simulink model "PassengerCar"  (R2019b)
settings: Solver=ode1  StartTime=0  StopTime=25  FixedStep=1.0000000000000000e-003  RelTol=1e-3
InitFcn:
  | sampleTime = str2double(get_param(bdroot, 'FixedStep'));
undefined symbols (not defined in the file or in its folder): AccPedalPos, BrakePedalPos, BrakeSwitch, DiscIntNeverNeededParam, DYNA4, EngSpd, IgnitionSwitch, InitialGear, InitialSpeed, IntendedEngTrq, LeftIndicator, MainBrakePress, MaxGear, MDL, MinGear, RefAcc, RefLane, RefLatPos, RefPath, RefPathCurv, RefSpd, RefSpdPreview, RefSpdRetrospect, RightIndicator, SteeringWheelAng, SteeringWheelTrq, UserDefinedRefValue, vm_const
libraries: UtilitiesLibrary x31, simulink x18, WheelSystemModules x13, LongitudinalControllerModules x13, LateralControllerModules x7, AnimationBusselectorModules x5, EnvironmentModules x5, BasicEngineControlModules x5, MiscellaneousControlModules x5, Animation3Modules x4, AuxiliariesModules x4, TireModules x4
(part 4 of 39)

== system PassengerCar/Traffic ==
  fromCTRL : Inport
  fromVehicle : Inport  Port=2
  DynaComponentInfo : Subsystem  Tag=DynaComponentInfo
      mask init:
      | data= get_param(gcb, 'UserData');
      settings: OpenFcn=DYNA4.ModelHandling.Component.ShowEditComponentInformationDialog(gcb);
      mask Display: disp(['Type = ', data.type, '\nGroup = ', data.group, '\nName = ', data.name ])
  Terminator : Terminator
  Terminator1 : Terminator
  TrafficOutputs : Subsystem
  Traffic : Outport  VectorParamsAs1DForOutWhenUnconnected=off
  wires:
  TrafficOutputs/1(Traffic) -> Traffic/1
  fromCTRL/1 -> Terminator/1
  fromVehicle/1 -> Terminator1/1

== system PassengerCar/Trailer ==
  fromCTRL : Inport
  fromVehicle : Inport  Port=2
  DynaComponentInfo : Subsystem  Tag=DynaComponentInfo
      mask init:
      | data= get_param(gcb, 'UserData');
      settings: OpenFcn=DYNA4.ModelHandling.Component.ShowEditComponentInformationDialog(gcb);
      mask Display: disp(['Type = ', data.type, '\nGroup = ', data.group, '\nName = ', data.name ])
  Terminator1 : Terminator
  Terminator4 : Terminator
  TrailerOutput : ReducedChassisModules/TrailerOutput  SystemSampleTime=-1  Latency=0  AutoFrameSizeCalculation=off
  Trailer : Outport  VectorParamsAs1DForOutWhenUnconnected=off
  wires:
  fromCTRL/1 -> Terminator4/1
  fromVehicle/1 -> Terminator1/1
  TrailerOutput/1 -> Trailer/1

== system PassengerCar/Vehicle ==
  fromCTRL : Inport
  fromTrailer : Inport  Port=2
  fromEnvironment : Inport  Port=3
  AnimationContentVehicle : Animation3Modules/AnimationContentVehicle  SystemSampleTime=-1  Latency=0  AutoFrameSizeCalculation=off
  Auxiliaries : Subsystem  Tag=vedynaEngineMask
  BrakeSystem : Subsystem  Tag=vedynaEngineMask
  Chassis : Subsystem  Tag=COMPONENT_CHASSIS
  CoolingSystem : Subsystem
  DriverInformationVehicle : DriverInformationModules/DriverInformationVehicle  DATA_NODE=MDL.Vehicle.DriverInformationVehicle  EngInrt=MDL.Vehicle.DriverInformationVehicle.EngInrt  OverallMass=MDL.Vehicle.DriverInformationVehicle.OverallMass  CoGPos=MDL.Vehicle.DriverInformationVehicle.CoGPos  FrontRearWheelBase=MDL.Vehicle.DriverInformationVehicle.FrontRearWheelBase  YawInrt=MDL.Vehicle.DriverInformationVehicle.YawInrt  FrontSteeringRatio=MDL.Vehicle.DriverInformationVehicle.FrontSteeringRatio  MaxLeftSteeringWheelAng=MDL.Vehicle.DriverInformationVehicle.MaxLeftSteeringWheelAng  MaxRightSteeringWheelAng=MDL.Vehicle.DriverInformationVehicle.MaxRightSteeringWheelAng  TransmissionType=MDL.Vehicle.DriverInformationVehicle.TransmissionType  NumFwdGears=MDL.Vehicle.DriverInformationVehicle.NumFwdGears  FrontTireUnloadedRadius=MDL.Vehicle.DriverInformationVehicle.FrontTireUnloadedRadius  RearTireUnloadedRadius=MDL.Vehicle.DriverInformationVehicle.RearTireUnloadedRadius  WheelRotAxisInrt=MDL.Vehicle.DriverInformationVehicle.WheelRotAxisInrt  MaxMainBrakePress=MDL.Vehicle.DriverInformationVehicle.MaxMainBrakePress  MaxDec=MDL.Vehicle.DriverInformationVehicle.MaxDec  LongAeroDragCoeff=MDL.Vehicle.DriverInformationVehicle.LongAeroDragCoeff  nShiftECU=MDL.Vehicle.DriverInformationVehicle.nShiftECU  FrontAxleLatStiff=MDL.Vehicle.DriverInformationVehicle.FrontAxleLatStiff  RearAxleLatStiff=MDL.Vehicle.DriverInformationVehicle.RearAxleLatStiff  EngTrqController=MDL.Vehicle.DriverInformationVehicle.EngTrqController
  Drivetrain : Subsystem  Tag=COMPONENT_DRIVETRAIN
  DynaComponentInfo : Subsystem  Tag=DynaComponentInfo
      mask init:
      | data= get_param(gcb, 'UserData');
      settings: OpenFcn=DYNA4.ModelHandling.Component.ShowEditComponentInformationDialog(gcb);
      mask Display: disp(['Type = ', data.type, '\nGroup = ', data.group, '\nName = ', data.name ])
  ElectricalSystem : Subsystem
  Engine : Subsystem  Tag=COMPONENT_ENGINE
  VehicleOutput : Subsystem  Tag=TESIS DYNAware Interface Block  mask{NeedsUpdate=off, SignalInfo=|}
      mask SignalInfo=|
      | {
      |   "Version": "4.6",
      |   "MuxedOutputBusName": "Vehicle",
      |   "MuxedInputBusName": "input",
      |   "MuxedInputSelected": false,
      |   "MuxedOutputSelected": true,
      |   "SignalData": [
      |     {
      |       "initialValue": "0.0",
      |       "name": "Auxiliaries",
      |       "comment": "",
      |       "minString": "",
      |       "maxString": "",
      |       "width": -1,
      |       "dataType": 0,
      |       "signalType": 1,
      |       "createSignal": false,
      |       "outputName": "Auxiliaries",
      |       "generateSignalAccessBlock": false,
      |       "accessId": "$(parentId).$(blockName).$(outputName)"
      |     },
      |     {
      |       "initialValue": "0.0",
      |       "name": "BrakeSystem",
      |       "comment": "",
      |       "minString": "",
      |       "maxString": "",
      |       "width": -1,
      |       "dataType": 0,
      |       "signalType": 1,
      |       "createSignal": false,
      |       "outputName": "BrakeSystem",
      |       "generateSignalAccessBlock": false,
      |       "accessId": "$(parentId).$(blockName).$(outputName)"
      |     },
      |     {
      |       "initialValue": "0.0",
      |       "name": "Chassis",
      |       "comment": "",
      |       "minString": "",
      |       "maxString": "",
      |       "width": -1,
      |       "dataType": 0,
      |       "signalType": 1,
      |       "createSignal": false,
      |       "outputName": "Chassis",
      |       "generateSignalAccessBlock": false,
      |       "accessId": "$(parentId).$(blockName).$(outputName)"
      |     },
      |     {
      |       "initialValue": "0.0",
      |       "name": "Drivetrain",
      |       "comment": "",
      |       "minString": "",
      |       "maxString": "",
      |       "width": -1,
      |       "dataType": 0,
      |       "signalType": 1,
      |       "createSignal": false,
      |       "outputName": "Drivetrain",
      |       "generateSignalAccessBlock": false,
      |       "accessId": "$(parentId).$(blockName).$(outputName)"
      |     },
      |     {
      |       "initialValue": "0.0",
      |       "name": "ElectricalSystem",
      |       "comment": "",
      |       "minString": "",
      |       "maxString": "",
      |       "width": -1,
      |       "dataType": 0,
      |       "signalType": 1,
      |       "createSignal": false,
      |       "outputName": "ElectricalSystem",
      |       "generateSignalAccessBlock": false,
      |       "accessId": "$(parentId).$(blockName).$(outputName)"
      |     },
      |     {
      |       "initialValue": "0.0",
      |       "name": "Engine",
      |       "comment": "",
      |       "minString": "",
      |       "maxString": "",
      |       "width": -1,
      |       "dataType": 0,
      |       "signalType": 1,
      |       "createSignal": false,
      |       "outputName": "Engine",
      |       "generateSignalAccessBlock": false,
      |       "accessId": "$(parentId).$(blockName).$(outputName)"
      |     },
      |     {
      |       "initialValue": "0.0",
      |       "name": "WheelSystem",
      |       "comment": "",
      |       "minString": "",
      |       "maxString": "",
      |       "width": -1,
      |       "dataType": 0,
      |       "signalType": 1,
      |       "createSignal": false,
      |       "outputName": "WheelSystem",
      |       "generateSignalAccessBlock": false,
      |       "accessId": "$(parentId).$(blockName).$(outputName)"
      |     },
      |     {
      |       "initialValue": "0.0",
      |       "name": "CoolingSystem",
      |       "comment": "",
      |       "minString": "",
      |       "maxString": "",
      |       "width": -1,
      |       "dataType": 0,
      |       "signalType": 1,
      |       "createSignal": false,
      |       "outputName": "CoolingSystem",
      |       "generateSignalAccessBlock": false,
      |       "accessId": "$(parentId).$(blockName).$(outputName)"
      |     },
      |     {
      |       "initialValue": "0.0",
      |       "name": "VehicleRoadInfo",
      |       "comment": "",
      |       "minString": "",
      |       "maxString": "",
      |       "width": -1,
      |       "dataType": 0,
      |       "signalType": 1,
      |       "createSignal": false,
      |       "outputName": "VehicleRoadInfo",
      |       "generateSignalAccessBlock": false,
      |       "accessId": "$(parentId).$(blockName).$(outputName)"
      |     },
      |     {
      |       "initialValue": "0.0",
      |       "name": "VehicleDriverInfo",
      |       "comment": "",
      |       "minString": "",
      |       "maxString": "",
      |       "width": -1,
      |       "dataType": 0,
      |       "signalType": 1,
      |       "createSignal": false,
      |       "outputName": "VehicleDriverInfo",
      |       "generateSignalAccessBlock": false,
      |       "accessId": "$(parentId).$(blockName).$(outputName)"
      |     }
      |   ]
      | }
      mask prompts: NeedsUpdate "Specify, if subsystem content needs to be updated"; SignalInfo "Signal Info (json)"
      mask help: DYNA4 Interface Block Version 4.6
      mask init:
      | blockName = get_param(gcbh, 'Name');
      | parentId = DYNA4.ModelHandling.AccessID.getFromHierarchy(gcbh);
      | TD.InterfaceBlock.ModelCallbacks.GenerateContent(gcb);
      settings: DeleteFcn=TD.InterfaceBlock.ModelCallbacks.CloseGUI( gcbh );  NameChangeFcn=TD.InterfaceBlock.ModelCallbacks.BlockRenamedHandler(gcbh);  OpenFcn=TD.InterfaceBlock.ModelCallbacks.OpenGUI( gcbh );  CloseFcn=TD.InterfaceBlock.ModelCallbacks.CloseGUI( gcbh );
      mask Display:
      | image('InterfaceBlock.png','center');
      | port_label('input',1, 'Auxiliaries');
      | port_label('input',2, 'BrakeSystem');
      | port_label('input',3, 'Chassis');
      | port_label('input',4, 'Drivetrain');
      | port_label('input',5, 'ElectricalSystem');
      | port_label('input',6, 'Engine');
      | port_label('input',7, 'WheelSystem');
      | port_label('input',8, 'CoolingSystem');
      | port_label('input',9, 'VehicleRoadInfo');
      | port_label('input',10, 'VehicleDriverInfo');
      | port_label('output',1, 'Vehicle');
  VehicleRoadInfo : Subsystem
  WheelSystem : Subsystem  Tag=COMPONENT_WHEELSYSTEM
  Vehicle : Outport  VectorParamsAs1DForOutWhenUnconnected=off
  wires:
  DriverInformationVehicle/1 -> VehicleOutput/10(VehicleDriverInfo___UNIQUE_1)
  VehicleRoadInfo/1(VehicleRoadInfo) -> VehicleOutput/9(VehicleRoadInfo___UNIQUE_1)
  CoolingSystem/1(CoolingSystem) -> VehicleOutput/8(CoolingSystem___UNIQUE_1)
  fromTrailer/1 -> Chassis/2(fromTrailer)
  fromEnvironment/1 -> CoolingSystem/6(fromEnvironment), Engine/2(fromEnvironment)
  fromCTRL/1 -> Auxiliaries/1(fromCTRL), Chassis/1(fromCTRL), Drivetrain/1(fromCTRL), ElectricalSystem/1(fromCTRL), DriverInformationVehicle/1, VehicleRoadInfo/1(fromCTRL), CoolingSystem/1(fromCTRL), WheelSystem/1(fromCTRL), Engine/1(fromCTRL), BrakeSystem/1(fromCTRL)
  ElectricalSystem/1(ElectricalSystem) -> CoolingSystem/5(fromElectricalSystem), Engine/5(fromElectricalSystem), Drivetrain/3(fromElectricalSystem), Auxiliaries/3(fromElectricalSystem), VehicleOutput/5(ElectricalSystem___UNIQUE_1)
  VehicleOutput/1(Vehicle___UNIQUE_1) -> Vehicle/1
  BrakeSystem/1(BrakeSystem) -> DriverInformationVehicle/2, WheelSystem/2(fromBrakeSystem), VehicleOutput/2(BrakeSystem___UNIQUE_1)
  Auxiliaries/1(Auxiliaries) -> ElectricalSystem/2(fromAuxiliaries), Drivetrain/2(fromAuxiliaries), VehicleOutput/1(Auxiliaries___UNIQUE_1)
  Chassis/1(Chassis) -> DriverInformationVehicle/3, VehicleRoadInfo/2(fromChassis), CoolingSystem/2(fromChassis), WheelSystem/3(fromChassis), Engine/3(fromChassis), BrakeSystem/2(fromChassis), VehicleOutput/3(Chassis___UNIQUE_1)
  Drivetrain/1(Drivetrain) -> Auxiliaries/2(fromDrivetrain), ElectricalSystem/3(fromDrivetrain), DriverInformationVehicle/4, CoolingSystem/4(fromDrivetrain), WheelSystem/4(fromDrivetrain), Engine/4(fromDrivetrain), VehicleOutput/4(Drivetrain___UNIQUE_1)
  WheelSystem/1(WheelSystem) -> DriverInformationVehicle/6, Drivetrain/5(fromWheelSystem), Chassis/4(fromWheelSystem), BrakeSystem/4(fromWheelSystem), VehicleOutput/7(WheelSystem___UNIQUE_1)
  Engine/1(Engine) -> DriverInformationVehicle/5, CoolingSystem/3(fromEngine), ElectricalSystem/4(fromEngine), Drivetrain/4(fromEngine), Chassis/3(fromEngine), Auxiliaries/4(fromEngine), BrakeSystem/3(fromEngine), VehicleOutput/6(Engine___UNIQUE_1)

== system PassengerCar/VehicleControl ==
  fromCTRL : Inport
  fromTrailer : Inport  Port=2
  fromVehicle : Inport  Port=3
  fromTraffic : Inport  Port=4
  DynaComponentInfo : Subsystem  Tag=DynaComponentInfo
      mask init:
      | data= get_param(gcb, 'UserData');
      settings: OpenFcn=DYNA4.ModelHandling.Component.ShowEditComponentInformationDialog(gcb);
      mask Display: disp(['Type = ', data.type, '\nGroup = ', data.group, '\nName = ', data.name ])
  InitialConditions : Subsystem
  LateralControl : Subsystem  VariantControlMode=Label  Variant=on  LabelModeActiveChoice=EnabledLateralControl
  LongitudinalControl : Subsystem
  Miscellaneous : Subsystem
  TraceMarker : UtilitiesLibrary/DYNA4 Trace Marker  Tag=DYNA4_TRACE_MARKER  SettingType=Standard  PrefixModelBlockID=on  PrefixRootSignalName=off  NamePattern='$(modelBlockID).$(rootSignalName)'
  VehicleControlInputs : Subsystem
  VehicleControlOutput : Subsystem  Tag=TESIS DYNAware Interface Block  mask{NeedsUpdate=off, SignalInfo=|}
      mask SignalInfo=|
      | {
      |   "Version": "4.6",
      |   "MuxedOutputBusName": "VehicleControl",
      |   "MuxedInputBusName": "fromLongitudinalControl",
      |   "MuxedInputSelected": false,
      |   "MuxedOutputSelected": true,
      |   "SignalData": [
      |     {
      |       "initialValue": "0.0",
      |       "name": "InitialConditions",
      |       "comment": "",
      |       "minString": "",
      |       "maxString": "",
      |       "width": -1,
      |       "dataType": 0,
      |       "signalType": 1,
      |       "createSignal": false,
      |       "outputName": "InitialConditions",
      |       "generateSignalAccessBlock": false,
      |       "accessId": "$(parentId).$(blockName).$(outputName)"
      |     },
      |     {
      |       "initialValue": "0.0",
      |       "name": "LongitudinalControl",
      |       "comment": "",
      |       "minString": "",
      |       "maxString": "",
      |       "width": -1,
      |       "dataType": 0,
      |       "signalType": 1,
      |       "createSignal": false,
      |       "outputName": "LongitudinalControl",
      |       "generateSignalAccessBlock": false,
      |       "accessId": "$(parentId).$(blockName).$(outputName)"
      |     },
      |     {
      |       "initialValue": "0.0",
      |       "name": "LateralControl",
      |       "comment": "",
      |       "minString": "",
      |       "maxString": "",
      |       "width": -1,
      |       "dataType": 0,
      |       "signalType": 1,
      |       "createSignal": false,
      |       "outputName": "LateralControl",
      |       "generateSignalAccessBlock": false,
      |       "accessId": "$(parentId).$(blockName).$(outputName)"
      |     },
      |     {
      |       "initialValue": "0.0",
      |       "name": "BrakeHydraulicsControl",
      |       "comment": "",
      |       "minString": "",
      |       "maxString": "",
      |       "width": -1,
      |       "dataType": 0,
      |       "signalType": 1,
      |       "createSignal": false,
      |       "outputName": "BrakeHydraulicsControl",
      |       "generateSignalAccessBlock": false,
      |       "accessId": "$(parentId).$(blockName).$(outputName)"
      |     },
      |     {
      |       "initialValue": "0.0",
      |       "name": "EngineControl",
      |       "comment": "",
      |       "minString": "",
      |       "maxString": "",
      |       "width": -1,
      |       "dataType": 0,
      |       "signalType": 1,
      |       "createSignal": false,
      |       "outputName": "EngineControl",
      |       "generateSignalAccessBlock": false,
      |       "accessId": "$(parentId).$(blockName).$(outputName)"
      |     },
      |     {
      |       "initialValue": "0.0",
      |       "name": "SuspensionTestRigControl",
      |       "comment": "",
      |       "minString": "",
      |       "maxString": "",
      |       "width": -1,
      |       "dataType": 0,
      |       "signalType": 1,
      |       "createSignal": false,
      |       "outputName": "SuspensionTestRigControl",
      |       "generateSignalAccessBlock": false,
      |       "accessId": "$(parentId).$(blockName).$(outputName)"
      |     },
      |     {
      |       "initialValue": "0.0",
      |       "name": "TemperatureControl",
      |       "comment": "",
      |       "minString": "",
      |       "maxString": "",
      |       "width": -1,
      |       "dataType": 0,
      |       "signalType": 1,
      |       "createSignal": false,
      |       "outputName": "TemperatureControl",
      |       "generateSignalAccessBlock": false,
      |       "accessId": "$(parentId).$(blockName).$(outputName)"
      |     },
      |     {
      |       "initialValue": "0.0",
      |       "name": "UserDefinedControl",
      |       "comment": "",
      |       "minString": "",
      |       "maxString": "",
      |       "width": -1,
      |       "dataType": 0,
      |       "signalType": 1,
      |       "createSignal": false,
      |       "outputName": "UserDefinedControl",
      |       "generateSignalAccessBlock": false,
      |       "accessId": "$(parentId).$(blockName).$(outputName)"
      |     }
      |   ]
      | }
      mask prompts: NeedsUpdate "Specify, if subsystem content needs to be updated"; SignalInfo "Signal Info (json)"
      mask help: DYNA4 Interface Block Version 4.6
      mask init:
      | blockName = get_param(gcbh, 'Name');
      | parentId = DYNA4.ModelHandling.AccessID.getFromHierarchy(gcbh);
      | TD.InterfaceBlock.ModelCallbacks.GenerateContent(gcb);
      settings: DeleteFcn=TD.InterfaceBlock.ModelCallbacks.CloseGUI( gcbh );  NameChangeFcn=TD.InterfaceBlock.ModelCallbacks.BlockRenamedHandler(gcbh);  OpenFcn=TD.InterfaceBlock.ModelCallbacks.OpenGUI( gcbh );  CloseFcn=TD.InterfaceBlock.ModelCallbacks.CloseGUI( gcbh );
      mask Display:
      | image('InterfaceBlock.png','center');
      | port_label('input',1, 'InitialConditions');
      | port_label('input',2, 'LongitudinalControl');
      | port_label('input',3, 'LateralControl');
      | port_label('input',4, 'BrakeHydraulicsControl');
      | port_label('input',5, 'EngineControl');
      | port_label('input',6, 'SuspensionTestRigControl');
      | port_label('input',7, 'TemperatureControl');
      | port_label('input',8, 'UserDefinedControl');
      | port_label('output',1, 'VehicleControl');
  VehicleControl : Outport  VectorParamsAs1DForOutWhenUnconnected=off
  wires:
  Miscellaneous/2(EngineControlParams) -> VehicleControlOutput/5(EngineControl___UNIQUE_1)
  Miscellaneous/5(UserDefinedControlParams) -> VehicleControlOutput/8(UserDefinedControl___UNIQUE_1)
  Miscellaneous/4(TemperatureControlParams) -> VehicleControlOutput/7(TemperatureControl___UNIQUE_1)
  Miscellaneous/3(SuspensionTestRigControlParams) -> VehicleControlOutput/6(SuspensionTestRigControl___UNIQUE_1)
  fromTraffic/1 -> VehicleControlInputs/4(fromTraffic)
  fromVehicle/1 -> VehicleControlInputs/2(fromVehicle)
  LongitudinalControl/1(LongitudinalControl) -> VehicleControlOutput/2(LongitudinalControl___UNIQUE_1)
  Miscellaneous/1(BrakeHydraulicsParams) -> VehicleControlOutput/4(BrakeHydraulicsControl___UNIQUE_1)
  LateralControl/1(LateralControl) -> VehicleControlOutput/3(LateralControl___UNIQUE_1)
  VehicleControlOutput/1(VehicleControl___UNIQUE_1) -> VehicleControl/1, TraceMarker/1
  fromCTRL/1 -> InitialConditions/1(fromCTRL), VehicleControlInputs/1(fromCTRL)
  VehicleControlInputs/1(SchedulerAbscissae) -> LateralControl/1(SchedulerAbscissae), LongitudinalControl/1(SchedulerAbscissae)
  VehicleControlInputs/2(CtrlSystemsAbscissae) -> Miscellaneous/1(Abscissae), LateralControl/2(CtrlSystemsAbscissae), LongitudinalControl/2(CtrlSystemsAbscissae)
  VehicleControlInputs/3(PhaseTerminationVals) -> LateralControl/3(PhaseTerminationVals), LongitudinalControl/3(PhaseTerminationVals)
  VehicleControlInputs/6(LongCTRL) -> LongitudinalControl/6(LongCTRL)
  VehicleControlInputs/4(VehicleInfo) -> LateralControl/4(VehicleInfo), LongitudinalControl/4(VehicleInfo)
  VehicleControlInputs/7(LongExtCtrlEnforced) -> LongitudinalControl/7(ExtCtrlVariablesEnforced)
  VehicleControlInputs/8(LongExtCtrlVals) -> LongitudinalControl/8(ExtCtrlVals)
  VehicleControlInputs/9(LatCTRL) -> LateralControl/5(LatCTRL)
  VehicleControlInputs/10(LatExtCtrlEnforced) -> LateralControl/6(ExtCtrlVariablesEnforced)
  VehicleControlInputs/11(LatExtCtrlVals) -> LateralControl/7(ExtCtrlVals)
  VehicleControlInputs/5(TrafficInfo) -> LongitudinalControl/5(TrafficInfo)
  fromTrailer/1 -> VehicleControlInputs/3(fromTrailer)
  InitialConditions/1(InitialConditions) -> VehicleControlOutput/1(InitialConditions___UNIQUE_1)

== system PassengerCar/Animation/DynaComponentInfo ==

== system PassengerCar/ControlUnits/ADAS ==
  fromCTRL : Inport
  fromVehicle : Inport  Port=2
  ADASOutput : Subsystem  Tag=TESIS DYNAware Interface Block  mask{NeedsUpdate=off, SignalInfo=|}
      mask SignalInfo=|
      | {
      |   "Version": "4.6",
      |   "MuxedOutputBusName": "ADAS",
      |   "MuxedInputBusName": "input",
      |   "MuxedInputSelected": false,
      |   "MuxedOutputSelected": true,
      |   "SignalData": [
      |     {
      |       "initialValue": "0.0",
      |       "name": "",
      |       "comment": "",
      |       "minString": "",
      |       "maxString": "",
      |       "width": 1,
      |       "dataType": 0,
      |       "signalType": 0,
      |       "createSignal": true,
      |       "outputName": "PrioritizedADASControl.LimitsActive[0;1]",
      |       "generateSignalAccessBlock": false,
      |       "accessId": "$(parentId).$(blockName).$(outputName)"
      |     },
      |     {
      |       "initialValue": "vm_const('PAR_NOT_GIVEN')",
      |       "name": "",
      |       "comment": "",
      |       "minString": "",
      |       "maxString": "",
      |       "width": 1,
      |       "dataType": 0,
      |       "signalType": 0,
      |       "createSignal": true,
      |       "outputName": "PrioritizedADASControl.UpperLimitTrq[Nm]",
      |       "generateSignalAccessBlock": false,
      |       "accessId": "$(parentId).$(blockName).$(outputName)"
      |     },
      |     {
      |       "initialValue": "-vm_const('PAR_NOT_GIVEN')",
      |       "name": "",
      |       "comment": "",
      |       "minString": "",
      |       "maxString": "",
      |       "width": 1,
      |       "dataType": 0,
      |       "signalType": 0,
      |       "createSignal": true,
      |       "outputName": "PrioritizedADASControl.LowerLimitTrq[Nm]",
      |       "generateSignalAccessBlock": false,
      |       "accessId": "$(parentId).$(blockName).$(outputName)"
      |     },
      |     {
      |       "initialValue": "0.0",
      |       "name": "",
      |       "comment": "",
      |       "minString": "",
      |       "maxString": "",
      |       "width": 1,
      |       "dataType": 0,
      |       "signalType": 0,
      |       "createSignal": true,
      |       "outputName": "PrioritizedADASControl.LowerLimitBrakePress[Pa]",
      |       "generateSignalAccessBlock": false,
      |       "accessId": "$(parentId).$(blockName).$(outputName)"
      |     },
      |     {
      |       "initialValue": "0.0",
      |       "name": "",
      |       "comment": "",
      |       "minString": "",
      |       "maxString": "",
      |       "width": 1,
      |       "dataType": 0,
      |       "signalType": 0,
      |       "createSignal": true,
      |       "outputName": "LongitudinalControlIntervention[0;1]",
      |       "generateSignalAccessBlock": false,
      |       "accessId": "$(parentId).$(blockName).$(outputName)"
      |     }
      |   ]
      | }
      mask prompts: NeedsUpdate "Specify, if subsystem content needs to be updated"; SignalInfo "Signal Info (json)"
      mask help: DYNA4 Interface Block Version 4.6
      mask init:
      | blockName = get_param(gcbh, 'Name');
      | parentId = DYNA4.ModelHandling.AccessID.getFromHierarchy(gcbh);
      | TD.InterfaceBlock.ModelCallbacks.GenerateContent(gcb);
      settings: DeleteFcn=TD.InterfaceBlock.ModelCallbacks.CloseGUI( gcbh );  NameChangeFcn=TD.InterfaceBlock.ModelCallbacks.BlockRenamedHandler(gcbh);  OpenFcn=TD.InterfaceBlock.ModelCallbacks.OpenGUI( gcbh );  CloseFcn=TD.InterfaceBlock.ModelCallbacks.CloseGUI( gcbh );
      settings: AttributesFormatString=|
      | PrioritizedADASControl.LimitsActive[0;1] = 0.0
      | PrioritizedADASControl.UpperLimitTrq[Nm] = vm_const('PAR_NOT_GIVEN')
      | PrioritizedADASControl.LowerLimitTrq[Nm] = -vm_const('PAR_NOT_GIVEN')
      | PrioritizedADASControl.LowerLimitBrakePress[Pa] = 0.0
      | ...
      mask Display:
      | image('InterfaceBlock.png','center');
      | port_label('output',1, 'ADAS');
  DynaComponentInfo : Subsystem  Tag=DynaComponentInfo
      mask init:
      | data= get_param(gcb, 'UserData');
      settings: OpenFcn=DYNA4.ModelHandling.Component.ShowEditComponentInformationDialog(gcb);
      mask Display: disp(['Type = ', data.type, '\nGroup = ', data.group, '\nName = ', data.name ])
  Terminator : Terminator
  Terminator1 : Terminator
  ADAS : Outport  VectorParamsAs1DForOutWhenUnconnected=off
  wires:
  ADASOutput/1(ADAS___UNIQUE_1) -> ADAS/1
  fromCTRL/1 -> Terminator/1
  fromVehicle/1 -> Terminator1/1

== system PassengerCar/ControlUnits/ControlUnitsOutput ==
  VCU___UNIQUE_1 : Inport  Description=|
      | <name>VCU</name>
      | <comment></comment>
  ADAS___UNIQUE_1 : Inport  Description=|  Port=2
      | <name>ADAS</name>
      | <comment></comment>
  LCU___UNIQUE_1 : Inport  Description=|  Port=3
      | <name>LCU</name>
      | <comment></comment>
  StateSensors___UNIQUE_1 : Inport  Description=|  Port=4
      | <name>StateSensors</name>
      | <comment></comment>
  __TDO__ControlUnits : BusCreator  Inputs=4
  ControlUnits___UNIQUE_1 : Outport  Description=|  VectorParamsAs1DForOutWhenUnconnected=off
      | <name>VCU</name>
      | <comment></comment>
  wires:
  VCU___UNIQUE_1/1 -> __TDO__ControlUnits/1  "VCU"
  ADAS___UNIQUE_1/1 -> __TDO__ControlUnits/2  "ADAS"
  LCU___UNIQUE_1/1 -> __TDO__ControlUnits/3  "LCU"
  StateSensors___UNIQUE_1/1 -> __TDO__ControlUnits/4  "StateSensors"
  __TDO__ControlUnits/1 -> ControlUnits___UNIQUE_1/1  "ControlUnits"

== system PassengerCar/ControlUnits/DynaComponentInfo ==

== system PassengerCar/ControlUnits/LCU ==
  fromCTRL : Inport
  fromVehicle : Inport  Port=2
  DynaComponentInfo : Subsystem  Tag=DynaComponentInfo
      mask init:
      | data= get_param(gcb, 'UserData');
      settings: OpenFcn=DYNA4.ModelHandling.Component.ShowEditComponentInformationDialog(gcb);
      mask Display: disp(['Type = ', data.type, '\nGroup = ', data.group, '\nName = ', data.name ])
  Generate Vehicle Light States : ControllerLibrary/Generate Vehicle Light States  minVelSwitchOn=50/3.6  minDecSwitchOn=6  maxDecSwitchOff=2.5  flashFrequency=5  flashDutyCycle=0.8  maxVelSwitchOnIndicators=1  indicatorFrequency=1.5  indicatorDutyCycle=0.5
  LCUOutput : Subsystem  Tag=TESIS DYNAware Interface Block  mask{NeedsUpdate=off, SignalInfo=|}
      mask SignalInfo=|
      | {
      |   "Version": "4.6",
      |   "MuxedOutputBusName": "LCU",
      |   "MuxedInputBusName": "input",
      |   "MuxedInputSelected": false,
      |   "MuxedOutputSelected": true,
      |   "SignalData": {
      |     "initialValue": "0.0",
      |     "name": "VehicleLights",
      |     "comment": "",
      |     "minString": "",
      |     "maxString": "",
      |     "width": -1,
      |     "dataType": 0,
      |     "signalType": 1,
      |     "createSignal": false,
      |     "outputName": "VehicleLights",
      |     "generateSignalAccessBlock": false,
      |     "accessId": "$(parentId).$(blockName).$(outputName)"
      |   }
      | }
      mask prompts: NeedsUpdate "Specify, if subsystem content needs to be updated"; SignalInfo "Signal Info (json)"
      mask help: DYNA4 Interface Block Version 4.6
      mask init:
      | blockName = get_param(gcbh, 'Name');
      | parentId = DYNA4.ModelHandling.AccessID.getFromHierarchy(gcbh);
      | TD.InterfaceBlock.ModelCallbacks.GenerateContent(gcb);
      settings: DeleteFcn=TD.InterfaceBlock.ModelCallbacks.CloseGUI( gcbh );  NameChangeFcn=TD.InterfaceBlock.ModelCallbacks.BlockRenamedHandler(gcbh);  OpenFcn=TD.InterfaceBlock.ModelCallbacks.OpenGUI( gcbh );  CloseFcn=TD.InterfaceBlock.ModelCallbacks.CloseGUI( gcbh );
      mask Display:
      | image('InterfaceBlock.png','center');
      | port_label('input',1, 'VehicleLights');
      | port_label('output',1, 'LCU');
  LCU : Outport  VectorParamsAs1DForOutWhenUnconnected=off
  wires:
  fromVehicle/1 -> Generate Vehicle Light States/2
  fromCTRL/1 -> Generate Vehicle Light States/1
  LCUOutput/1(LCU___UNIQUE_1) -> LCU/1
  Generate Vehicle Light States/1 -> LCUOutput/1(VehicleLights___UNIQUE_1)

== system PassengerCar/ControlUnits/StateSensors ==
  fromCTRL : Inport
  fromTrailer : Inport  Port=2
  fromVehicle : Inport  Port=3
  fromTraffic : Inport  Port=4
  DynaComponentInfo : Subsystem  Tag=DynaComponentInfo
      mask init:
      | data= get_param(gcb, 'UserData');
      settings: OpenFcn=DYNA4.ModelHandling.Component.ShowEditComponentInformationDialog(gcb);
      mask Display: disp(['Type = ', data.type, '\nGroup = ', data.group, '\nName = ', data.name ])
  InertialMeasurementUnit : StateSensorModules/InertialMeasurementUnit  DATA_NODE=MDL.ControlUnits.StateSensors.InertialMeasurementUnit  SensorPosition=MDL.ControlUnits.StateSensors.InertialMeasurementUnit.SensorPosition  SensorOrientation=MDL.ControlUnits.StateSensors.InertialMeasurementUnit.SensorOrientation  EnableGeoCoordinates=MDL.ControlUnits.StateSensors.InertialMeasurementUnit.EnableGeoCoordinates
  StateSensorsOutput : Subsystem  Tag=TESIS DYNAware Interface Block  mask{NeedsUpdate=off, SignalInfo=|}
      mask SignalInfo=|
      | {
      |   "Version": "4.6",
      |   "MuxedOutputBusName": "StateSensors",
      |   "MuxedInputBusName": "input",
      |   "MuxedInputSelected": false,
      |   "MuxedOutputSelected": true,
      |   "SignalData": {
      |     "initialValue": "0.0",
      |     "name": "IMU",
      |     "comment": "",
      |     "minString": "",
      |     "maxString": "",
      |     "width": -1,
      |     "dataType": 0,
      |     "signalType": 1,
      |     "createSignal": false,
      |     "outputName": "IMU",
      |     "generateSignalAccessBlock": false,
      |     "accessId": "$(parentId).$(blockName).$(outputName)"
      |   }
      | }
      mask prompts: NeedsUpdate "Specify, if subsystem content needs to be updated"; SignalInfo "Signal Info (json)"
      mask help: DYNA4 Interface Block Version 4.6
      mask init:
      | blockName = get_param(gcbh, 'Name');
      | parentId = DYNA4.ModelHandling.AccessID.getFromHierarchy(gcbh);
      | TD.InterfaceBlock.ModelCallbacks.GenerateContent(gcb);
      settings: DeleteFcn=TD.InterfaceBlock.ModelCallbacks.CloseGUI( gcbh );  NameChangeFcn=TD.InterfaceBlock.ModelCallbacks.BlockRenamedHandler(gcbh);  OpenFcn=TD.InterfaceBlock.ModelCallbacks.OpenGUI( gcbh );  CloseFcn=TD.InterfaceBlock.ModelCallbacks.CloseGUI( gcbh );
      mask Display:
      | image('InterfaceBlock.png','center');
      | port_label('input',1, 'IMU');
      | port_label('output',1, 'StateSensors');
  Terminator : Terminator
  Terminator1 : Terminator
  Terminator2 : Terminator
  StateSensors : Outport  VectorParamsAs1DForOutWhenUnconnected=off
  wires:
  fromVehicle/1 -> InertialMeasurementUnit/1
  StateSensorsOutput/1(StateSensors___UNIQUE_1) -> StateSensors/1
  InertialMeasurementUnit/1 -> StateSensorsOutput/1(IMU___UNIQUE_1)
  fromCTRL/1 -> Terminator/1
  fromTraffic/1 -> Terminator1/1
  fromTrailer/1 -> Terminator2/1

== system PassengerCar/ControlUnits/VCU ==
  fromCTRL : Inport
  fromVehicle : Inport  Port=2
  fromADAS : Inport  Port=3
  ADASInterface : VCULibrary/ADASInterface  SystemSampleTime=-1  Latency=0  AutoFrameSizeCalculation=off
  DynaComponentInfo : Subsystem  Tag=DynaComponentInfo
      mask init:
      | data= get_param(gcb, 'UserData');
      settings: OpenFcn=DYNA4.ModelHandling.Component.ShowEditComponentInformationDialog(gcb);
      mask Display: disp(['Type = ', data.type, '\nGroup = ', data.group, '\nName = ', data.name ])
  InputFromADAS : Subsystem  Tag=TESIS DYNAware Interface Block  mask{NeedsUpdate=off, SignalInfo=|}
      mask SignalInfo=|
      | {
      |   "Version": "4.6",
      |   "MuxedOutputBusName": "PrioritizedADASControl",
      |   "MuxedInputBusName": "fromADAS",
      |   "MuxedInputSelected": true,
      |   "MuxedOutputSelected": true,
      |   "SignalData": {
      |     "initialValue": "0.0",
      |     "name": "PrioritizedADASControl",
      |     "comment": "",
      |     "minString": "",
      |     "maxString": "",
      |     "width": -1,
      |     "dataType": 0,
      |     "signalType": 1,
      |     "createSignal": false,
      |     "outputName": "PrioritizedADASControl",
      |     "generateSignalAccessBlock": false,
      |     "accessId": "$(parentId).$(blockName).$(outputName)"
      |   }
      | }
      mask prompts: NeedsUpdate "Specify, if subsystem content needs to be updated"; SignalInfo "Signal Info (json)"
      mask help: DYNA4 Interface Block Version 4.6
      mask init:
      | blockName = get_param(gcbh, 'Name');
      | parentId = DYNA4.ModelHandling.AccessID.getFromHierarchy(gcbh);
      | TD.InterfaceBlock.ModelCallbacks.GenerateContent(gcb);
      settings: DeleteFcn=TD.InterfaceBlock.ModelCallbacks.CloseGUI( gcbh );  NameChangeFcn=TD.InterfaceBlock.ModelCallbacks.BlockRenamedHandler(gcbh);  OpenFcn=TD.InterfaceBlock.ModelCallbacks.OpenGUI( gcbh );  CloseFcn=TD.InterfaceBlock.ModelCallbacks.CloseGUI( gcbh );
      mask Display:
      | image('InterfaceBlock.png','center');
      | port_label('input',1, 'fromADAS');
      | port_label('output',1, 'PrioritizedADASControl');
  InputFromCTRL : Subsystem  Tag=TESIS DYNAware Interface Block  mask{NeedsUpdate=off, SignalInfo=|}
      mask SignalInfo=|
      | {
      |   "Version": "4.6",
      |   "MuxedOutputBusName": "Drivetrain",
      |   "MuxedInputBusName": "fromCTRL",
      |   "MuxedInputSelected": true,
      |   "MuxedOutputSelected": false,
      |   "SignalData": [
      |     {
      |       "initialValue": "0.0",
      |       "name": "CTRL.LongitudinalControl.AccPedalPos[0_1]",
      |       "comment": "Accelerator pedal position",
      |       "minString": "",
      |       "maxString": "",
      |       "width": 1,
      |       "dataType": 0,
      |       "signalType": 0,
      |       "createSignal": false,
      |       "outputName": "AccPedalPos[0_1]",
      |       "generateSignalAccessBlock": false,
      |       "accessId": "$(parentId).$(blockName).$(outputName)"
      |     },
      |     {
      |       "initialValue": "0.0",
      |       "name": "CTRL.LongitudinalControl.BrakePedalPos[0_1]",
      |       "comment": "",
      |       "minString": "",
      |       "maxString": "",
      |       "width": -1,
      |       "dataType": 0,
      |       "signalType": 0,
      |       "createSignal": false,
      |       "outputName": "BrakePedalPos[0_1]",
      |       "generateSignalAccessBlock": false,
      |       "accessId": "$(parentId).$(blockName).$(outputName)"
      |     },
      |     {
      |       "initialValue": "0.0",
      |       "name": "CTRL.LongitudinalControl.DriverInfo.MeanEngMaxTrq[Nm]",
      |       "comment": "",
      |       "minString": "",
      |       "maxString": "",
      |       "width": 1,
      |       "dataType": 0,
      |       "signalType": 0,
      |       "createSignal": false,
      |       "outputName": "MeanEngMaxTrq[Nm]",
      |       "generateSignalAccessBlock": false,
      |       "accessId": "$(parentId).$(blockName).$(outputName)"
      |     },
      |     {
      |       "initialValue": "0.0",
      |       "name": "CTRL.LongitudinalControl.DriverInfo.MeanEngDragTrq[Nm]",
      |       "comment": "",
      |       "minString": "",
      |       "maxString": "",
      |       "width": 1,
      |       "dataType": 0,
      |       "signalType": 0,
      |       "createSignal": false,
      |       "outputName": "MeanEngDragTrq[Nm]",
      |       "generateSignalAccessBlock": false,
      |       "accessId": "$(parentId).$(blockName).$(outputName)"
      |     },
      |     {
      |       "initialValue": "0.0",
      |       "name": "CTRL.LongitudinalControl.DriverInfo.ThirtyPercentAccPedalEngTrq[Nm]",
      |       "comment": "",
      |       "minString": "",
      |       "maxString": "",
      |       "width": 1,
      |       "dataType": 0,
      |       "signalType": 0,
      |       "createSignal": false,
      |       "outputName": "ThirtyPercentAccPedalEngTrq[Nm]",
      |       "generateSignalAccessBlock": false,
      |       "accessId": "$(parentId).$(blockName).$(outputName)"
      |     }
      |   ]
      | }
      mask prompts: NeedsUpdate "Specify, if subsystem content needs to be updated"; SignalInfo "Signal Info (json)"
      mask help: DYNA4 Interface Block Version 4.6
      mask init:
      | blockName = get_param(gcbh, 'Name');
      | parentId = DYNA4.ModelHandling.AccessID.getFromHierarchy(gcbh);
      | TD.InterfaceBlock.ModelCallbacks.GenerateContent(gcb);
      settings: DeleteFcn=TD.InterfaceBlock.ModelCallbacks.CloseGUI( gcbh );  NameChangeFcn=TD.InterfaceBlock.ModelCallbacks.BlockRenamedHandler(gcbh);  OpenFcn=TD.InterfaceBlock.ModelCallbacks.OpenGUI( gcbh );  CloseFcn=TD.InterfaceBlock.ModelCallbacks.CloseGUI( gcbh );
      mask Display:
      | image('InterfaceBlock.png','center');
      | port_label('input',1, 'fromCTRL');
      | port_label('output',1, 'AccPedalPos[0_1]');
      | port_label('output',2, 'BrakePedalPos[0_1]');
      | port_label('output',3, 'MeanEngMaxTrq[Nm]');
      | port_label('output',4, 'MeanEngDragTrq[Nm]');
      | port_label('output',5, 'ThirtyPercentAccPedalEngTrq[Nm]');
  InputFromVehicle : Subsystem  Tag=TESIS DYNAware Interface Block  mask{NeedsUpdate=off, SignalInfo=|}
      mask SignalInfo=|
      | {
      |   "Version": "4.6",
      |   "MuxedOutputBusName": "Drivetrain",
      |   "MuxedInputBusName": "fromVehicle",
      |   "MuxedInputSelected": true,
      |   "MuxedOutputSelected": false,
      |   "SignalData": {
      |     "initialValue": "0.0",
      |     "name": "BrakeSystem.BrakeSystemPhysics.MaxMainBrakePress[Pa]",
      |     "comment": "Maximum main brake pressure",
      |     "minString": "",
      |     "maxString": "",
      |     "width": 1,
      |     "dataType": 0,
      |     "signalType": 0,
      |     "createSignal": false,
      |     "outputName": "MaxMainBrakePress[Pa]",
      |     "generateSignalAccessBlock": false,
      |     "accessId": "$(parentId).$(blockName).$(outputName)"
      |   }
      | }
      mask prompts: NeedsUpdate "Specify, if subsystem content needs to be updated"; SignalInfo "Signal Info (json)"
      mask help: DYNA4 Interface Block Version 4.6
      mask init:
      | blockName = get_param(gcbh, 'Name');
      | parentId = DYNA4.ModelHandling.AccessID.getFromHierarchy(gcbh);
      | TD.InterfaceBlock.ModelCallbacks.GenerateContent(gcb);
      settings: DeleteFcn=TD.InterfaceBlock.ModelCallbacks.CloseGUI( gcbh );  NameChangeFcn=TD.InterfaceBlock.ModelCallbacks.BlockRenamedHandler(gcbh);  OpenFcn=TD.InterfaceBlock.ModelCallbacks.OpenGUI( gcbh );  CloseFcn=TD.InterfaceBlock.ModelCallbacks.CloseGUI( gcbh );
      mask Display:
      | image('InterfaceBlock.png','center');
      | port_label('input',1, 'fromVehicle');
      | port_label('output',1, 'MaxMainBrakePress[Pa]');
  TransmissionLoad : VCULibrary/TransmissionLoad  SystemSampleTime=-1  Latency=0  AutoFrameSizeCalculation=off
  VCUOutput : Subsystem  Tag=TESIS DYNAware Interface Block  mask{NeedsUpdate=off, SignalInfo=|}
      mask SignalInfo=|
      | {
      |   "Version": "4.6",
      |   "MuxedOutputBusName": "VCU",
      |   "MuxedInputBusName": "input",
      |   "MuxedInputSelected": false,
      |   "MuxedOutputSelected": true,
      |   "SignalData": [
      |     {
      |       "initialValue": "0.0",
      |       "name": "TransmissionLoad[0_1]",
      |       "comment": "",
      |       "minString": "",
      |       "maxString": "",
      |       "width": 1,
      |       "dataType": 0,
      |       "signalType": 0,
      |       "createSignal": false,
      |       "outputName": "TransmissionLoad[0_1]",
      |       "generateSignalAccessBlock": false,
      |       "accessId": "$(parentId).$(blockName).$(outputName)"
      |     },
      |     {
      |       "initialValue": "0.0",
      |       "name": "IntendedEngTrq[Nm]",
      |       "comment": "Intended torque of engine",
      |       "minString": "",
      |       "maxString": "",
      |       "width": 1,
      |       "dataType": 0,
      |       "signalType": 0,
      |       "createSignal": false,
      |       "outputName": "IntendedEngTrq[Nm]",
      |       "generateSignalAccessBlock": false,
      |       "accessId": "$(parentId).$(blockName).$(outputName)"
      |     },
      |     {
      |       "initialValue": "0.0",
      |       "name": "IntendedEngTrqActive[0;1]",
      |       "comment": "",
      |       "minString": "",
      |       "maxString": "",
      |       "width": 1,
      |       "dataType": 0,
      |       "signalType": 0,
      |       "createSignal": false,
      |       "outputName": "IntendedEngTrqActive[0;1]",
      |       "generateSignalAccessBlock": false,
      |       "accessId": "$(parentId).$(blockName).$(outputName)"
      |     },
      |     {
      |       "initialValue": "0.0",
      |       "name": "IntendedMainBrakePress[Pa]",
      |       "comment": "",
      |       "minString": "",
      |       "maxString": "",
      |       "width": 1,
      |       "dataType": 0,
      |       "signalType": 0,
      |       "createSignal": false,
      |       "outputName": "IntendedMainBrakePress[Pa]",
      |       "generateSignalAccessBlock": false,
      |       "accessId": "$(parentId).$(blockName).$(outputName)"
      |     },
      |     {
      |       "initialValue": "0.0",
      |       "name": "IntendedMainBrakePressActive[0;1]",
      |       "comment": "",
      |       "minString": "",
      |       "maxString": "",
      |       "width": 1,
      |       "dataType": 0,
      |       "signalType": 0,
      |       "createSignal": false,
      |       "outputName": "IntendedMainBrakePressActive[0;1]",
      |       "generateSignalAccessBlock": false,
      |       "accessId": "$(parentId).$(blockName).$(outputName)"
      |     },
      |     {
      |       "initialValue": "0.0",
      |       "name": "",
      |       "comment": "Driving state",
      |       "minString": "",
      |       "maxString": "",
      |       "width": 1,
      |       "dataType": 0,
      |       "signalType": 0,
      |       "createSignal": true,
      |       "outputName": "DrivingState[-]",
      |       "generateSignalAccessBlock": false,
      |       "accessId": "$(parentId).$(blockName).$(outputName)"
      |     },
      |     {
      |       "initialValue": "1.0",
      |       "name": "",
      |       "comment": "",
      |       "minString": "",
      |       "maxString": "",
      |       "width": 1,
      |       "dataType": 0,
      |       "signalType": 0,
      |       "createSignal": true,
      |       "outputName": "DriverInfo.ConventionalVehicleSwitch[0;1]",
      |       "generateSignalAccessBlock": false,
      |       "accessId": "$(parentId).$(blockName).$(outputName)"
      |     },
      |     {
      |       "initialValue": "1.0",
      |       "name": "",
      |       "comment": "",
      |       "minString": "0",
      |       "maxString": "1",
      |       "width": 1,
      |       "dataType": 0,
      |       "signalType": 0,
      |       "createSignal": true,
      |       "outputName": "EngRunPermission[0;1]",
      |       "generateSignalAccessBlock": false,
      |       "accessId": "$(parentId).$(blockName).$(outputName)"
      |     }
      |   ]
      | }
      mask prompts: NeedsUpdate "Specify, if subsystem content needs to be updated"; SignalInfo "Signal Info (json)"
      mask help: DYNA4 Interface Block Version 4.6
      mask init:
      | blockName = get_param(gcbh, 'Name');
      | parentId = DYNA4.ModelHandling.AccessID.getFromHierarchy(gcbh);
      | TD.InterfaceBlock.ModelCallbacks.GenerateContent(gcb);
      settings: DeleteFcn=TD.InterfaceBlock.ModelCallbacks.CloseGUI( gcbh );  NameChangeFcn=TD.InterfaceBlock.ModelCallbacks.BlockRenamedHandler(gcbh);  OpenFcn=TD.InterfaceBlock.ModelCallbacks.OpenGUI( gcbh );  CloseFcn=TD.InterfaceBlock.ModelCallbacks.CloseGUI( gcbh );
      settings: AttributesFormatString=|
      | DrivingState[-] = 0.0
      | DriverInfo.ConventionalVehicleSwitch[0;1] = 1.0
      | EngRunPermission[0;1] = 1.0
      mask Display:
      | image('InterfaceBlock.png','center');
      | port_label('input',1, 'TransmissionLoad[0_1]');
      | port_label('input',2, 'IntendedEngTrq[Nm]');
      | port_label('input',3, 'IntendedEngTrqActive[0;1]');
      | port_label('input',4, 'IntendedMainBrakePress[Pa]');
      | port_label('input',5, 'IntendedMainBrakePressActive[0;1]');
      | port_label('output',1, 'VCU');
  VCU : Outport  VectorParamsAs1DForOutWhenUnconnected=off
  wires:
  InputFromCTRL/2(BrakePedalPos[0_1]___UNIQUE_1) -> ADASInterface/2
  InputFromVehicle/1(MaxMainBrakePress[Pa]___UNIQUE_1) -> ADASInterface/6
  InputFromCTRL/1(AccPedalPos[0_1]) -> ADASInterface/1
  fromVehicle/1 -> InputFromVehicle/1(fromVehicle)
  fromCTRL/1 -> InputFromCTRL/1(fromCTRL)
  fromADAS/1 -> InputFromADAS/1(fromADAS)
  VCUOutput/1(VCU___UNIQUE_1) -> VCU/1
  ADASInterface/1 -> TransmissionLoad/2, VCUOutput/2(IntendedEngTrq[Nm]___UNIQUE_1)
  InputFromADAS/1(PrioritizedADASControl___UNIQUE_1) -> ADASInterface/7
  ADASInterface/2 -> VCUOutput/3(IntendedEngTrqActive[0;1]___UNIQUE_1)
  ADASInterface/3 -> VCUOutput/4(IntendedMainBrakePress[Pa]___UNIQUE_1)
  ADASInterface/4 -> VCUOutput/5(IntendedMainBrakePressActive[0;1]___UNIQUE_1)
  TransmissionLoad/1 -> VCUOutput/1(TransmissionLoad[0_1]___UNIQUE_1)
  InputFromCTRL/5(ThirtyPercentAccPedalEngTrq[Nm]___UNIQUE_1) -> ADASInterface/5
  InputFromCTRL/3(MeanEngMaxTrq[Nm]___UNIQUE_1) -> TransmissionLoad/1, ADASInterface/3
  InputFromCTRL/4(MeanEngDragTrq[Nm]___UNIQUE_1) -> ADASInterface/4

== system PassengerCar/Environment/DynaComponentInfo ==

== system PassengerCar/Environment/EnvironmentOutput ==
  WindImpact___UNIQUE_1 : Inport  Description=|
      | <name>WindImpact</name>
      | <comment></comment>
  RoadFrictionScaling___UNIQUE_1 : Inport  Description=|  Port=2
      | <name>RoadFrictionScaling</name>
      | <comment></comment>
  AdditionalRoadElevation___UNIQUE_1 : Inport  Description=|  Port=3
      | <name>AdditionalRoadElevation</name>
      | <comment></comment>
  AmbientConditions___UNIQUE_1 : Inport  Description=|  Port=4
      | <name>AmbientConditions</name>
      | <comment></comment>
  __TDO__Environment : BusCreator  Inputs=4
  Environment___UNIQUE_1 : Outport  Description=|  VectorParamsAs1DForOutWhenUnconnected=off
      | <name>WindImpact</name>
      | <comment></comment>
  wires:
  WindImpact___UNIQUE_1/1 -> __TDO__Environment/1  "WindImpact"
  RoadFrictionScaling___UNIQUE_1/1 -> __TDO__Environment/2  "RoadFrictionScaling"
  AdditionalRoadElevation___UNIQUE_1/1 -> __TDO__Environment/3  "AdditionalRoadElevation"
  AmbientConditions___UNIQUE_1/1 -> __TDO__Environment/4  "AmbientConditions"
  __TDO__Environment/1 -> Environment___UNIQUE_1/1  "Environment"

== system PassengerCar/Environment/Road ==
  DynaSystemInfo : Subsystem  Tag=DynaSystemInfo
      mask init:
      | data = get_param(gcb, 'UserData');
      settings: OpenFcn=DYNA4.ModelHandling.System.ShowEditSystemInformationDialog(gcb);
      mask Display: disp(['System Name = ', data.name])
  Road : RoadModules/3DRoad  DATA_NODE=MDL.Environment.Road

== system PassengerCar/SimulationControl/DynaComponentInfo ==

== system PassengerCar/Traffic/DynaComponentInfo ==
